simulink model "fullModelRefPWM"  (R2022b)
settings: Solver=ode15s  StartTime=0.0  StopTime=2  RelTol=1e-3  EnableMultiTasking=on
PreLoadFcn:
  | load allParamValues.mat
libraries: SignalEditorBlockLib x1
settings Model: Creator=jrivitus  LastModifiedBy=bensweet
settings SolverCC: MaxConsecutiveZCs=25  AlgebraicLoopSolver=TrustRegion  MaxZcPerStep=1
settings DataIOCC: LimitDataPoints=on  SaveFormat=Array  ReturnWorkspaceOutputs=off
settings OptimizationCC: DefaultParameterBehavior=Inlined  ExpressionDepthLimit=2147483647  InitFltsAndDblsToZero=on  LifeSpan=inf
settings DebuggingCC: UnconnectedInputMsg=warning  UnconnectedOutputMsg=warning  UnconnectedLineMsg=warning  PregeneratedLibrarySubsystemCodeDiagnostic=none  SFMachineParentedDataDiag=warning
settings HardwareCC: ProdBitPerPointer=32  ProdBitPerSizeT=32  ProdBitPerPtrDiffT=32  ProdLargestAtomicFloat=None  ProdIntDivRoundTo=Undefined  ProdEndianess=Unspecified  ProdWordSize=32  ProdHWDeviceType=32-bit Generic
settings ModelReferenceCC: EnableRefExpFcnMdlSchedulingChecks=on  ModelReferenceMinAlgLoopOccurrences=on  PropagateSignalLabelsOutOfModel=off
settings SFSimCC: SimUseLocalCustomCode=off
settings RTWCC: RTWUseLocalCustomCode=off  DLArmComputeVersion=19.05
settings CodeAppCC: StateflowObjectComments=on
settings GRTTargetCC: TargetLangStandard=C89/C90 (ANSI)  CombineOutputUpdateFcns=off  GRTInterface=on
settings ConfigComp: CovMetricSettings=dw  CovSaveCumulativeToWorkspaceVar=on  CovSaveSingleToWorkspaceVar=on  CovExternalEMLEnable=off  CovSFcnEnable=off

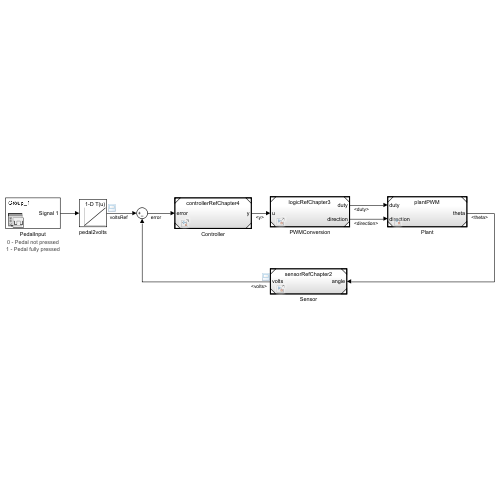
[thumbnail: Simulink's stored preview of the top-level diagram]
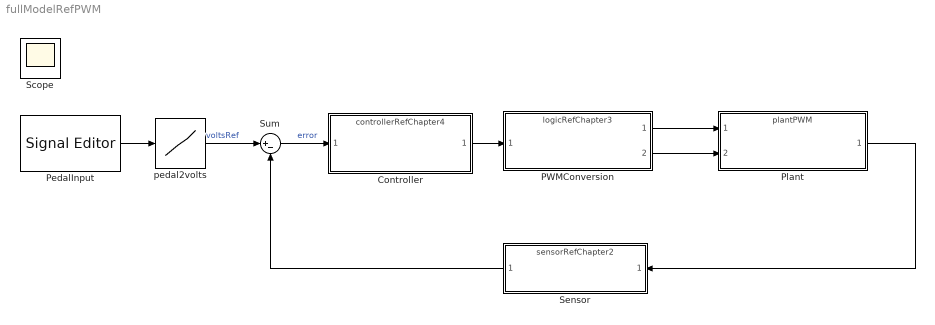
== system fullModelRefPWM ==
  Controller : ModelReference  ModelNameDialog=controllerRefChapter4  SimulationMode=Normal  ModelReferenceVersion=6.0
  PWMConversion : ModelReference  ModelNameDialog=logicRefChapter3  SimulationMode=Normal  ModelReferenceVersion=5.0
  PedalInput : SignalEditorBlockLib/Signal Editor  FileName=fullModelRefPWM_PedalInput_dataset.mat  ActiveScenario=Group_1  ActiveSignal=Signal 1  IsBus=off  OutputBusObjectStr=Bus: BusObject  SampleTime=0  OutputAfterFinalValue=Extrapolation  Unit=inherit  PreserveSignalName=on
      settings: AttributesFormatString=0 - Pedal not pressed\n1 - Pedal fully pressed
  Plant : ModelReference  ModelNameDialog=plantPWM  SimulationMode=Normal  ModelReferenceVersion=5.0
  Sensor : ModelReference  ModelNameDialog=sensorRefChapter2  SimulationMode=Normal  ModelReferenceVersion=5.0
  Sum : Sum  Inputs=|+-
  pedal2volts : Lookup_n-D  NumberOfTableDimensions=1  BreakpointsForDimension1=[0 1]  Table=[0.5 4.5]  RndMeth=Simplest
  Scope : Scope
  wires:
  PedalInput/1 -> pedal2volts/1
  pedal2volts/1 -> Sum/1  "voltsRef"
  Sum/1 -> Controller/1  "error"
  Controller/1 -> PWMConversion/1
  PWMConversion/1 -> Plant/1
  PWMConversion/2 -> Plant/2
  Plant/1 -> Sensor/1
  Sensor/1 -> Sum/2
